simulink model "hw4simulink"  (R2023a)
settings: Solver=VariableStepAuto  StartTime=0.0  StopTime=100  RelTol=1e-3
values from neighbouring files (symbols this model uses):
  w0 = param.w0    [HW3.m]    (also in HW4.m)
libraries: slpidlib x1, simulink x1
settings Model: Creator=enson  LastModifiedBy=enson

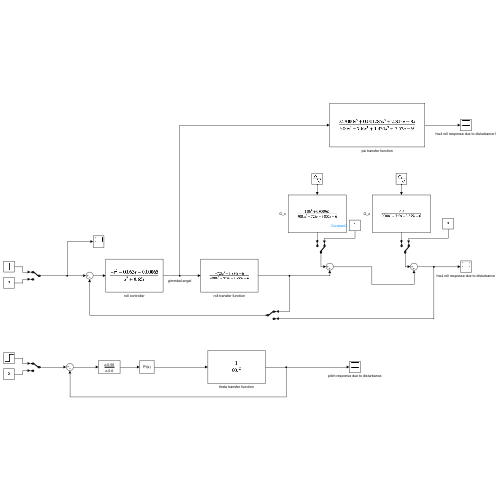
[thumbnail: Simulink's stored preview of the top-level diagram]
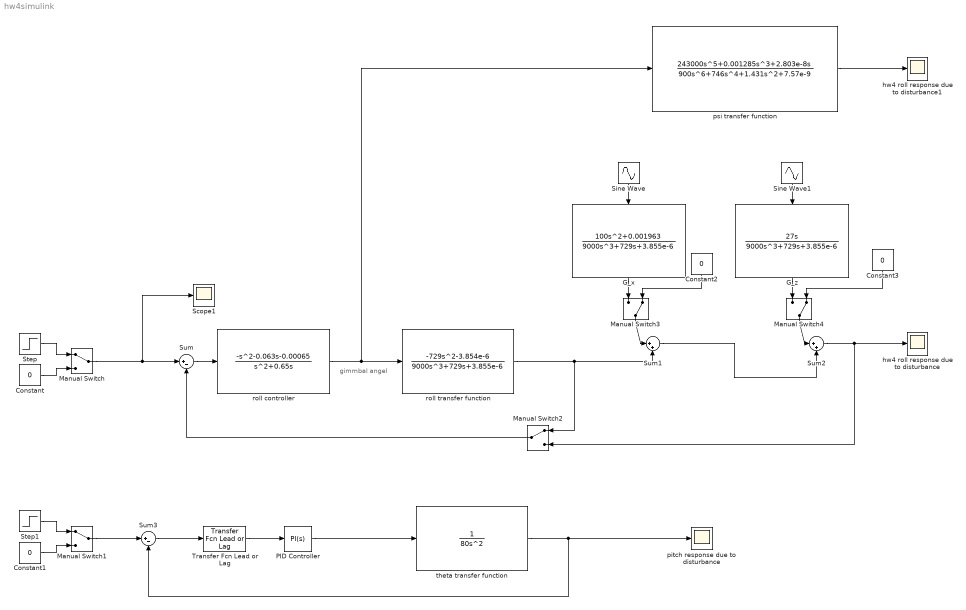
== system hw4simulink ==
  note: gimmbal angel
  Constant{,1..3} (4 alike) : Constant  Value=0
  G_x : TransferFcn  Numerator=[100 0 0.001963]  Denominator=[9000 0 729 3.855e-6]
  G_z : TransferFcn  Numerator=[27 0]  Denominator=[9000 0 729 3.855e-6]
  Manual Switch : ManualSwitch
  Manual Switch1 : ManualSwitch
  Manual Switch2 : ManualSwitch
  Manual Switch3 : ManualSwitch  CurrentSetting=0
  Manual Switch4 : ManualSwitch  CurrentSetting=0
  PID Controller : slpidlib/PID Controller  Controller=PI  Form=Ideal  TimeDomain=Continuous-time  UseExternalTs=off  SampleTime=-1  IntegratorMethod=Forward Euler  FilterMethod=Forward Euler  ControllerParametersSource=internal  P=0.810494359328635  I=0.00183266204715948  UseKiTs=off  D=0  N=100  UseFilter=on  TunerSelectOption=Transfer Function Based (PID Tuner App)  InitialConditionSource=internal  InitialConditionForIntegrator=0  InitialConditionForFilter=0  DifferentiatorICPrevScaledInput=0  ExternalReset=none  TrackingMode=off  Kt=1  LimitOutput=off  SatLimitsSource=internal  UpperSaturationLimit=inf  LowerSaturationLimit=-inf  LinearizeAsGain=on  AntiWindupMode=none  Kb=1  LimitIntegrator=off  UpperIntegratorSaturationLimit=inf  LowerIntegratorSaturationLimit=-inf  POutMin=[]  POutMax=[]  IOutMin=[]  IOutMax=[]  DOutMin=[]  DOutMax=[]  NOutMin=[]  NOutMax=[]  SumOutMin=[]  SumOutMax=[]  SaturationOutMin=[]  SaturationOutMax=[]  PParamMin=[]  PParamMax=[]  IParamMin=[]  IParamMax=[]  DParamMin=[]  DParamMax=[]  NParamMin=[]  NParamMax=[]  KbParamMin=[]  KbParamMax=[]  KtParamMin=[]  KtParamMax=[]  KbOutMin=[]  KbOutMax=[]  KtOutMin=[]  KtOutMax=[]  IntegratorOutMin=[]  IntegratorOutMax=[]  FilterOutMin=[]  FilterOutMax=[]  SumI1OutMin=[]  SumI1OutMax=[]  SumI2OutMin=[]  SumI2OutMax=[]  SumI3OutMin=[]  SumI3OutMax=[]  SumI4OutMin=[]  SumI4OutMax=[]  SumDOutMin=[]  SumDOutMax=[]  DifferentiatorOutMin=[]  DifferentiatorOutMax=[]  FilterDiffOutCoefMin=[]  FilterDiffOutCoefMax=[]  ReciprocalOutMin=[]  ReciprocalOutMax=[]  SumDenOutMin=[]  SumDenOutMax=[]  SumNumOutMin=[]  SumNumOutMax=[]  DivideOutMin=[]  DivideOutMax=[]  UdiffTsProdOutMin=[]  UdiffTsProdOutMax=[]  NTsProdOutMin=[]  NTsProdOutMax=[]  UintegralTsProdOutMin=[]  UintegralTsProdOutMax=[]  UngainTsProdOutMin=[]  UngainTsProdOutMax=[]  ClampingZeroOutDataTypeStr=Inherit: Inherit via back propagation  ClampingZeroOutMin=[]  ClampingZeroOutMax=[]  FilterDenConstantOutDataTypeStr=Inherit: Inherit via back propagation  FilterDenConstantOutMin=[]  FilterDenConstantOutMax=[]  PCopyOutDataTypeStr=Inherit: Inherit via back propagation  PCopyOutMin=[]  PCopyOutMax=[]  NCopyOutDataTypeStr=Inherit: Inherit via back propagation  NCopyOutMin=[]  NCopyOutMax=[]  IntegratorContinuousStateAttributes=''  IntegratorStateMustResolveToSignalObject=off  IntegratorRTWStateStorageClass=Auto  FilterContinuousStateAttributes=''  FilterStateMustResolveToSignalObject=off  FilterRTWStateStorageClass=Auto  ParallelPVariant=Passthrough  IdealPVariant=InternalParameters  IVariant=InternalParameters  DVariant=Disabled  IntegratorVariant=Continuous  SatVariant=Disabled  AWVariant=Passthrough  PCopyVariant=Disabled  TRVariant=Disabled  FdbkBlocksVariant=Forward  IdealPFdbkVariant=Disabled  SatFdbkVariant=Disabled  DerivativeFilterVariant=Disabled  NVariant=Disabled  NCopyVariant=Disabled_SignalSpec  FilterICVariant=Disabled  IntegratorICVariant=InternalICs  ExternalResetVariant=Disabled  TRSumVariant=Passthrough  SumFdbkVariant=Disabled  SumVariant=Sum_PI  TsampFilterVariant=InternalTs  TsampNgainVariant=Passthrough  TsampIntegralVariant=Disabled_SignalSpec  ExternalSaturationOutDataTypeStr=Inherit: Same as second input
  Scope1 : Scope
  Sine Wave : Sin  Amplitude=10e-4  Bias=10e-5  Frequency=w0  SampleTime=0
  Sine Wave1 : Sin  Amplitude=10e-4  Bias=10e-5  Frequency=w0  SampleTime=0
  Step : Step  Before=deg2rad(5)  After=deg2rad(5)  SampleTime=0
  Step1 : Step  Before=deg2rad(5)  After=deg2rad(5)  SampleTime=0
  Sum : Sum  Inputs=|+-
  Sum1 : Sum  Inputs=|++
  Sum2 : Sum  Inputs=|++
  Sum3 : Sum  Inputs=|+-
  Transfer Fcn Lead or Lag : simulink/Discrete/Transfer Fcn Lead or Lag  PoleZ=0.6  ZeroZ=0.56  ICPrevOutput=0.0  ICPrevInput=0.0  DoSatur=off
  hw4 roll response due to disturbance : Scope
  hw4 roll response due to disturbance1 : Scope
  pitch response due to disturbance : Scope
  psi transfer function : TransferFcn  Numerator=[243000 0 0.001285 0 2.803e-8 0]  Denominator=[900 0 746 0 1.431 0 7.57e-9]
  roll controller : TransferFcn  Numerator=[-1 -0.063 -0.00065]  Denominator=[1 0.65,0]
  roll transfer function : TransferFcn  Numerator=[-729 0 -3.854e-6]  Denominator=[9000 0 729 3.855e-6]
  theta transfer function : TransferFcn  Denominator=[80 0 0]
  wires:
  roll controller/1 -> psi transfer function/1, roll transfer function/1
  Sum/1 -> roll controller/1
  roll transfer function/1 -> Manual Switch2/1, Sum1/2
  Sum1/1 -> Sum2/2
  Sum2/1 -> Manual Switch2/2, hw4 roll response due to disturbance/1
  Sine Wave/1 -> G_x/1
  Sine Wave1/1 -> G_z/1
  psi transfer function/1 -> hw4 roll response due to disturbance1/1
  Step/1 -> Manual Switch/1
  Manual Switch/1 -> Scope1/1, Sum/1
  Constant/1 -> Manual Switch/2
  Step1/1 -> Manual Switch1/1
  Constant1/1 -> Manual Switch1/2
  Manual Switch2/1 -> Sum/2
  G_x/1 -> Manual Switch3/1
  G_z/1 -> Manual Switch4/1
  Manual Switch3/1 -> Sum1/1
  Manual Switch4/1 -> Sum2/1
  Constant2/1 -> Manual Switch3/2
  Constant3/1 -> Manual Switch4/2
  PID Controller/1 -> theta transfer function/1
  theta transfer function/1 -> Sum3/2, pitch response due to disturbance/1
  Sum3/1 -> Transfer Fcn Lead or Lag/1
  Manual Switch1/1 -> Sum3/1
  Transfer Fcn Lead or Lag/1 -> PID Controller/1
